simulink library "Lib_PF_BusGenDC_TMATS"  (R2017a)
settings: Solver=ode45  StartTime=0.0  StopTime=10.0  RelTol=1e-3  EnableMultiTasking=on
Description:
  | Thomas Modules
settings Model: Creator=jwchapm2  LastModifiedBy=glthoma1
settings DataIOCC: LimitDataPoints=on  SaveFormat=Array
settings OptimizationCC: ExpressionDepthLimit=2147483647  LifeSpan=inf
settings DebuggingCC: UnderspecifiedInitializationDetection=Classic  MergeDetectMultiDrivingBlocksExec=none  SolverPrmCheckMsg=warning  StateNameClashWarn=warning  SFUnexpectedBacktrackingDiag=warning  SFNoUnconditionalDefaultTransitionDiag=warning  SFExecutionAtInitializationDiag=none
settings HardwareCC: ProdBitPerPointer=32  ProdBitPerSizeT=32  ProdBitPerPtrDiffT=32  ProdLargestAtomicFloat=None  ProdIntDivRoundTo=Undefined  ProdEndianess=Unspecified  ProdWordSize=32  ProdHWDeviceType=32-bit Generic
settings ModelReferenceCC: PropagateSignalLabelsOutOfModel=off
settings GRTTargetCC: TargetLangStandard=C89/C90 (ANSI)  GeneratePreprocessorConditionals=Disable all
settings ConfigComp: CovMetricSettings=dw  CovHtmlReporting=on  CovSaveCumulativeToWorkspaceVar=on  CovSaveSingleToWorkspaceVar=on  CovExternalEMLEnable=off

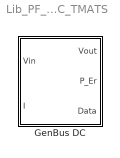
== system Lib_PF_BusGenDC_TMATS ==
  GenBus DC : Subsystem  mask{PeInEN_M=off, P_M=2, BlkNm_M=double(gcb)}
      mask prompts: PeInEN_M "PeInEN_M - External Pelec"; P_M "P_M - generated real power"; BlkNm_M "Block name as double for simulink output"
      mask init:
      | %Manage Power Inputs
      | if PeInEN_M == 1
      |     if strcmp(get_param([BlkNm_M '/Pelec'],'BlockType'),'Constant')
      |         MSK_ReplaceBlock_TMATS([BlkNm_M '/Pelec'],'built-in/Inport');
      |     end
      |     set_param([BlkNm_M '/Pelec'],'Port',num2str(2));
      | elseif PeInEN_M == 0
      |     if strcmp(get_param([BlkNm_M '/Pelec'],'BlockType'),'Inport')
      |         MSK_ReplaceBlock_TMATS([BlkNm_M '/Pelec'],'built-in/Constant');
      |         set_param([BlkNm_M '/Pelec'],'Value','P_M');
      |     end
      | end
      mask Callback PeInEN_M: MSK_SEC_Enables_TMATS('PeInEN_M',2,'dis')

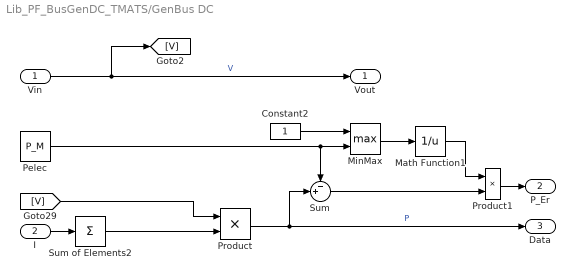
== system Lib_PF_BusGenDC_TMATS/GenBus DC ==
  Vin : Inport
  I : Inport  Port=2
  Constant2 : Constant
  Math Function1 : Math  Operator=reciprocal  SaturateOnIntegerOverflow=on
  MinMax : MinMax  Function=max  Inputs=2
  Pelec : Constant  Value=P_M
  Product : Product
  Product1 : Product
  Sum : Sum  Inputs=-+|
  Sum of Elements2 : Sum  Inputs=+
  Vout : Outport
  P_Er : Outport  Port=2
  Data : Outport  Port=3
  wires:
  Sum of Elements2/1 -> Product/2
  [V] -> Product/1
  I/1 -> Sum of Elements2/1
  Product/1 -> Data/1, Sum/2  "P"
  Vin/1 -> Vout/1, [V]  "V"
  Sum/1 -> Product1/2
  Pelec/1 -> MinMax/2, Sum/1
  Constant2/1 -> MinMax/1
  MinMax/1 -> Math Function1/1
  Math Function1/1 -> Product1/1
  Product1/1 -> P_Er/1
